simulink model "hb_llc_close_loop"  (R2024a)
settings: Solver=ode4  StartTime=0.0  StopTime=0.01  FixedStep=1e-08  RelTol=1e-3
libraries: spsCurrentMeasurementLib x7, spsVoltageMeasurementLib x7, spsSeriesRLCBranchLib x5, spsDiodeLib x4, spsMosfetLib x4, spsDCVoltageSourceLib x1, spsLinearTransformerLib x1, slpidlib x1, spsPWMGeneratorDCDCLib x1, sps_lib x1
settings Model: Creator=aditigupta  LastModifiedBy=aditigupta

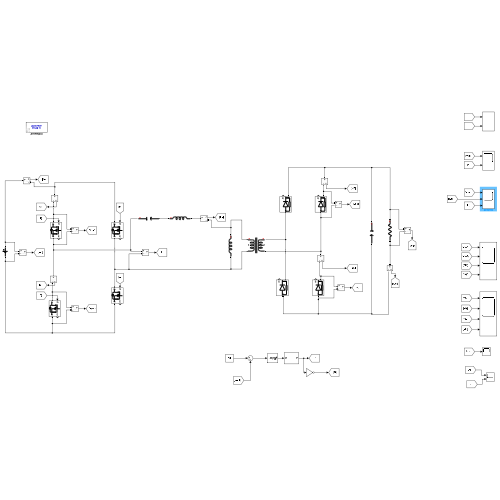
[thumbnail: Simulink's stored preview of the top-level diagram]
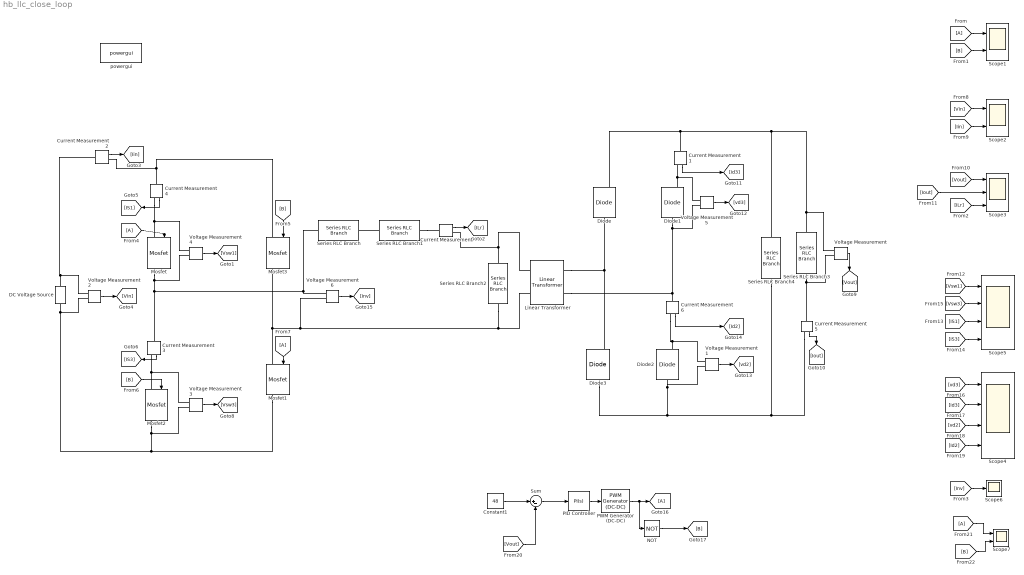
== system hb_llc_close_loop ==
  Constant1 : Constant  Value=48
  Current Measurement{,1..6} (7 alike) : spsCurrentMeasurementLib/Current Measurement  PhasorSimulation=off  OutputType=Complex  PSBequivalent=0
  DC Voltage Source : spsDCVoltageSourceLib/DC Voltage Source  Amplitude=400  Measurements=None
  Diode{,1..3} (4 alike) : spsDiodeLib/Diode  Ron=0.001  Lon=0  Vf=0.8  IC=0  UseSnubber=0  Rs=500  Cs=250e-9  Measurements=on
  From{,4,7,21} (4 alike) : From
  Goto16 : Goto
  Linear Transformer : spsLinearTransformerLib/Linear Transformer  UNITS=pu  NominalPower=[ 1000 100e3 ]  winding1=[ 8.33 0 0]  winding2=[1 0 0 ]  ThreeWindings=off  winding3=[ 315e3 0.002 0.08 ]  RmLm=[ 500 500 ]  Measurements=None  DataType=off
  Mosfet{,1..3} (4 alike) : spsMosfetLib/Mosfet  Ron=0.1  Lon=0  Rd=0.01  Vfd=0  IC=0  Rs=1e5  Cs=inf  Measurements=on
  NOT : Logic  Operator=NOT  IconShape=distinctive  AllPortsSameDT=off  OutDataTypeStr=boolean
  PID Controller : slpidlib/PID Controller  Controller=PI  Form=Parallel  TimeDomain=Continuous-time  UseExternalTs=off  SampleTime=-1  IntegratorMethod=Forward Euler  FilterMethod=Forward Euler  ControllerParametersSource=internal  P=0.00765  I=105.51  UseKiTs=off  D=0  UseExternalDerivativeSource=off  N=100  UseFilter=on  TunerSelectOption=Transfer Function Based (PID Tuner App)  InitialConditionSource=internal  InitialConditionForIntegrator=0  InitialConditionForFilter=0  DifferentiatorICPrevScaledInput=0  ExternalReset=none  TrackingMode=off  Kt=1  LimitOutput=on  SatLimitsSource=internal  UpperSaturationLimit=1  LowerSaturationLimit=0  LinearizeAsGain=on  AntiWindupMode=clamping  Kb=1  LimitIntegrator=off  UpperIntegratorSaturationLimit=inf  LowerIntegratorSaturationLimit=-inf  POutMin=[]  POutMax=[]  IOutMin=[]  IOutMax=[]  DOutMin=[]  DOutMax=[]  NOutMin=[]  NOutMax=[]  SumOutMin=[]  SumOutMax=[]  SaturationOutMin=[]  SaturationOutMax=[]  PParamMin=[]  PParamMax=[]  IParamMin=[]  IParamMax=[]  DParamMin=[]  DParamMax=[]  NParamMin=[]  NParamMax=[]  KbParamMin=[]  KbParamMax=[]  KtParamMin=[]  KtParamMax=[]  KbOutMin=[]  KbOutMax=[]  KtOutMin=[]  KtOutMax=[]  IntegratorOutMin=[]  IntegratorOutMax=[]  FilterOutMin=[]  FilterOutMax=[]  SumI1OutMin=[]  SumI1OutMax=[]  SumI2OutMin=[]  SumI2OutMax=[]  SumI3OutMin=[]  SumI3OutMax=[]  SumI4OutMin=[]  SumI4OutMax=[]  SumDOutMin=[]  SumDOutMax=[]  DifferentiatorOutMin=[]  DifferentiatorOutMax=[]  FilterDiffOutCoefMin=[]  FilterDiffOutCoefMax=[]  ReciprocalOutMin=[]  ReciprocalOutMax=[]  SumDenOutMin=[]  SumDenOutMax=[]  SumNumOutMin=[]  SumNumOutMax=[]  DivideOutMin=[]  DivideOutMax=[]  UdiffTsProdOutMin=[]  UdiffTsProdOutMax=[]  NTsProdOutMin=[]  NTsProdOutMax=[]  UintegralTsProdOutMin=[]  UintegralTsProdOutMax=[]  UngainTsProdOutMin=[]  UngainTsProdOutMax=[]  ClampingZeroOutDataTypeStr=Inherit: Inherit via back propagation  ClampingZeroOutMin=[]  ClampingZeroOutMax=[]  FilterDenConstantOutDataTypeStr=Inherit: Inherit via back propagation  FilterDenConstantOutMin=[]  FilterDenConstantOutMax=[]  PCopyOutDataTypeStr=Inherit: Inherit via back propagation  PCopyOutMin=[]  PCopyOutMax=[]  NCopyOutDataTypeStr=Inherit: Inherit via back propagation  NCopyOutMin=[]  NCopyOutMax=[]  IntegratorContinuousStateAttributes=''  IntegratorStateMustResolveToSignalObject=off  IntegratorRTWStateStorageClass=Auto  FilterContinuousStateAttributes=''  FilterStateMustResolveToSignalObject=off  FilterRTWStateStorageClass=Auto  ParallelPVariant=InternalParameters  IdealPVariant=Disabled  IVariant=InternalParameters  DVariant=Disabled  IntegratorVariant=Continuous  SatVariant=Enabled  AWVariant=ContClampingParallel  PCopyVariant=Disabled  TRVariant=Disabled  FdbkBlocksVariant=Forward  IdealPFdbkVariant=Disabled  SatFdbkVariant=Disabled  DerivativeFilterVariant=Disabled  NVariant=Disabled  NCopyVariant=Disabled_SignalSpec  FilterICVariant=Disabled  IntegratorICVariant=InternalICs  ExternalResetVariant=Disabled  TRSumVariant=Passthrough  SumFdbkVariant=Disabled  SumVariant=Sum_PI  TsampFilterVariant=InternalTs  TsampNgainVariant=Passthrough  TsampIntegralVariant=Disabled_SignalSpec  ExternalSaturationOutDataTypeStr=Inherit: Same as second input  DerivativeSourceVariant=Disabled
  PWM Generator (DC-DC) : spsPWMGeneratorDCDCLib/PWM Generator (DC-DC)  Fsw=100000  Ts=0
  Scope1 : Scope  NumInputPorts=2
  Scope2 : Scope  NumInputPorts=2
  Scope3 : Scope  NumInputPorts=3
  Scope4 : Scope  NumInputPorts=4
  Scope5 : Scope  NumInputPorts=4
  Scope6 : Scope
  Scope7 : Scope  NumInputPorts=2
  Series RLC Branch : spsSeriesRLCBranchLib/Series RLC Branch  LConnTagsString=__new0  RConnTagsString=__new0  BranchType=C  Resistance=1  Inductance=1e-3  SetiL0=off  InitialCurrent=0  Capacitance=0.030e-6  Setx0=off  InitialVoltage=0  Measurements=None
  Series RLC Branch1 : spsSeriesRLCBranchLib/Series RLC Branch  LConnTagsString=__new0  RConnTagsString=__new0  BranchType=L  Resistance=1  Inductance=82.616e-6  SetiL0=off  InitialCurrent=0  Capacitance=1e-6  Setx0=off  InitialVoltage=0  Measurements=None
  Series RLC Branch2 : spsSeriesRLCBranchLib/Series RLC Branch  LConnTagsString=__new0  RConnTagsString=__new0  BranchType=L  Resistance=1  Inductance=5.2*82.616e-6  SetiL0=off  InitialCurrent=0  Capacitance=1e-6  Setx0=off  InitialVoltage=0  Measurements=None
  Series RLC Branch3 : spsSeriesRLCBranchLib/Series RLC Branch  LConnTagsString=__new0  RConnTagsString=__new0  BranchType=R  Resistance=2.304  Inductance=1e-3  SetiL0=off  InitialCurrent=0  Capacitance=1e-6  Setx0=off  InitialVoltage=0  Measurements=None
  Series RLC Branch4 : spsSeriesRLCBranchLib/Series RLC Branch  LConnTagsString=__new0  RConnTagsString=__new0  BranchType=C  Resistance=2.592  Inductance=1e-3  SetiL0=off  InitialCurrent=0  Capacitance=2e-6  Setx0=off  InitialVoltage=0  Measurements=None
  Sum : Sum  Inputs=|+-
  Voltage Measurement{,1..6} (7 alike) : spsVoltageMeasurementLib/Voltage Measurement  PhasorSimulation=off  OutputType=Complex  PSBequivalent=0
  powergui : sps_lib/powergui  Priority=1  SimulationMode=Discrete  SampleTime=1/100000000  frequency=60  Iterations=50  frequencyindice=0  Pbase=100e6  ErrMax=1e-4  UnitsV=kV  UnitsW=MW  buscounter=0  FunctionMessages=off  echomessages=off  EnableUseOfTLC=off  CurrentSourceSwitches=off  DisableSnubberDevices=off  DisableRonSwitches=off  DisableVfSwitches=off  DisplayEquations=off  AutomaticDiscreteSolvers=off  SolverType=Tustin/Backward Euler (TBE)  Interpol=off  ExternalGateDelay=off  methode=off  Ts=100  x0status=blocks  SPID=on  SwTol=0  HookPort=off  NonlinearTolerance=1e-4  nMaxIteration=100  ContinueOnMaxIteration=off  RestoreLinks=warning  ResistiveCurrentMeasurement=off  Frange=[0:2:500]  Ylog=off  Xlog=on  ShowGrid=off  save=off  variable=ZData  structure=0  ZoomFFT=off  StartTime=0.0  cycles=1  DisplayStyle=1  fundamental=60  FreqAxis=off  MaxFrequency=1000  frequencyindicesteady=1  RmsSteady=1  display=off
  wires:
  [B] -> Mosfet3/1
  [B] -> Mosfet2/1
  From7/1 -> Mosfet1/1
  Current Measurement/1 -> [ILr]
  Current Measurement2/1 -> [Iin]
  Voltage Measurement2/1 -> [Vin]
  From4/1 -> Mosfet/1
  Current Measurement3/1 -> [IS3]
  Current Measurement4/1 -> [IS1]
  Voltage Measurement4/1 -> [Vsw1]
  Voltage Measurement3/1 -> [Vsw3]
  [B] -> Scope1/2
  From/1 -> Scope1/1
  [Vin] -> Scope2/1
  [Iin] -> Scope2/2
  Voltage Measurement/1 -> [Vout]
  Current Measurement5/1 -> [Iout]
  [Vout] -> Scope3/1
  [Iout] -> Scope3/2
  [ILr] -> Scope3/3
  [Vsw1] -> Scope5/1
  [Vsw3] -> Scope5/2
  [IS1] -> Scope5/3
  Current Measurement1/1 -> [id3]
  Voltage Measurement5/1 -> [vd3]
  Voltage Measurement1/1 -> [vd2]
  Current Measurement6/1 -> [Id2]
  [Id2] -> Scope4/4
  [vd2] -> Scope4/3
  [id3] -> Scope4/2
  [vd3] -> Scope4/1
  [IS3] -> Scope5/4
  Voltage Measurement6/1 -> [Inv]
  [Inv] -> Scope6/1
  Sum/1 -> PID Controller/1
  PID Controller/1 -> PWM Generator (DC-DC)/1
  [Vout] -> Sum/2
  PWM Generator (DC-DC)/1 -> NOT/1, Goto16/1
  Constant1/1 -> Sum/1
  NOT/1 -> [B]
  From21/1 -> Scope7/1
  [B] -> Scope7/2
  connections:
  Mosfet1/LConn1 -- Voltage Measurement6/LConn2 -- Linear Transformer/LConn2 -- Series RLC Branch2/RConn1 -- Mosfet3/RConn1
  DC Voltage Source/RConn1 -- Voltage Measurement2/LConn1 -- Current Measurement2/LConn1
  Mosfet/LConn1 -- Current Measurement4/RConn1 -- Voltage Measurement4/LConn1
  DC Voltage Source/LConn1 -- Voltage Measurement3/LConn2 -- Mosfet2/RConn1 -- Mosfet1/RConn1 -- Voltage Measurement2/LConn2
  Mosfet2/LConn1 -- Current Measurement3/RConn1 -- Voltage Measurement3/LConn1
  Current Measurement2/RConn1 -- Mosfet3/LConn1 -- Current Measurement4/LConn1
  Mosfet/RConn1 -- Series RLC Branch/LConn1 -- Voltage Measurement6/LConn1 -- Current Measurement3/LConn1 -- Voltage Measurement4/LConn2
  Series RLC Branch1/LConn1 -- Series RLC Branch/RConn1
  Series RLC Branch1/RConn1 -- Current Measurement/LConn1
  Diode1/LConn1 -- Linear Transformer/RConn2 -- Current Measurement6/LConn1 -- Voltage Measurement5/LConn2
  Diode3/LConn1 -- Voltage Measurement1/LConn2 -- Diode2/LConn1 -- Series RLC Branch4/RConn1 -- Current Measurement5/RConn1
  Series RLC Branch3/LConn1 -- Current Measurement1/LConn1 -- Diode/RConn1 -- Series RLC Branch4/LConn1 -- Voltage Measurement/LConn1
  Diode/LConn1 -- Diode3/RConn1 -- Linear Transformer/RConn1
  Series RLC Branch2/LConn1 -- Linear Transformer/LConn1 -- Current Measurement/RConn1
  Series RLC Branch3/RConn1 -- Voltage Measurement/LConn2 -- Current Measurement5/LConn1
  Diode1/RConn1 -- Voltage Measurement5/LConn1 -- Current Measurement1/RConn1
  Voltage Measurement1/LConn1 -- Current Measurement6/RConn1 -- Diode2/RConn1
